simulink model "ContinuousTimeModelling"  (R2021b)
settings: Solver=VariableStepAuto  StartTime=0.0  StopTime=10.0  RelTol=1e-3
libraries: simulink x1
settings Model: Creator=randy  LastModifiedBy=randy

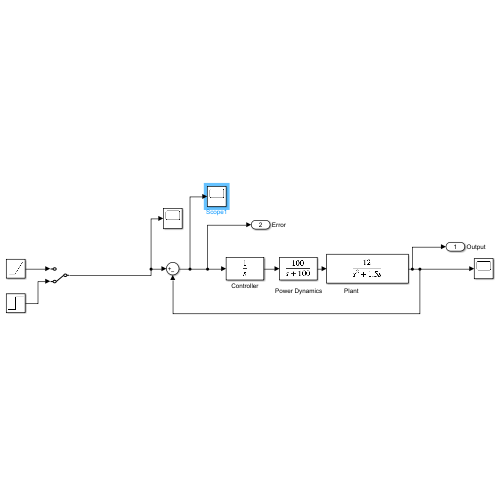
[thumbnail: Simulink's stored preview of the top-level diagram]
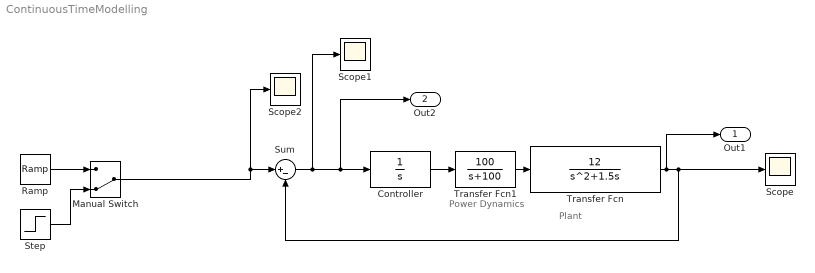
== system ContinuousTimeModelling ==
  note: Power Dynamics
  note: Plant
  Controller : TransferFcn  Denominator=[1 0 ]
  Manual Switch : ManualSwitch  CurrentSetting=0
  Ramp : simulink/Sources/Ramp  slope=1  start=0  InitialOutput=0
  Scope : Scope
  Scope1 : Scope
  Scope2 : Scope
  Step : Step  After=58  SampleTime=0
  Sum : Sum  Inputs=|+-
  Transfer Fcn : TransferFcn  Numerator=[12]  Denominator=[1 1.5 0 ]
  Transfer Fcn1 : TransferFcn  Numerator=[100 ]  Denominator=[1 100]
  Out1 : Outport  SignalName=Output
  Out2 : Outport  Port=2  SignalName=Error
  wires:
  Manual Switch/1 -> Scope2/1, Sum/1
  Transfer Fcn/1 -> Scope/1, Sum/2, Out1/1
  Sum/1 -> Scope1/1, Controller/1, Out2/1
  Transfer Fcn1/1 -> Transfer Fcn/1
  Controller/1 -> Transfer Fcn1/1
  Step/1 -> Manual Switch/2
  Ramp/1 -> Manual Switch/1
